simulink model "gm_sampleModel1552_5_sub"  (R2023a)
settings: Solver=VariableStepAuto  StartTime=0.0  StopTime=10.0  RelTol=1e-3
libraries: simulink x2
settings Model: Creator=user1  LastModifiedBy=user1
settings OptimizationCC: BlockReduction=off  ConditionallyExecuteInputs=off
settings DebuggingCC: InheritedTsInSrcMsg=none

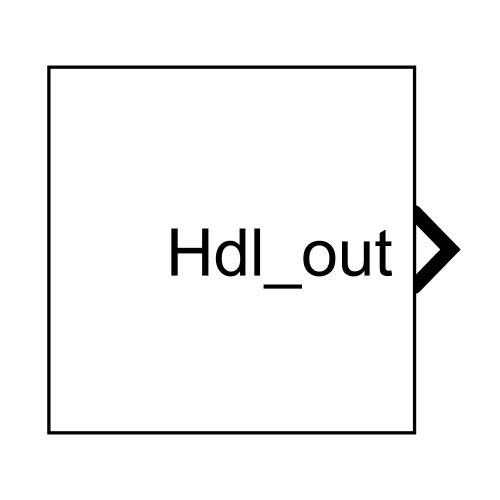
[thumbnail: Simulink's stored preview of the top-level diagram]
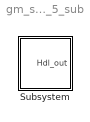
== system gm_sampleModel1552_5_sub ==
  Subsystem : Subsystem

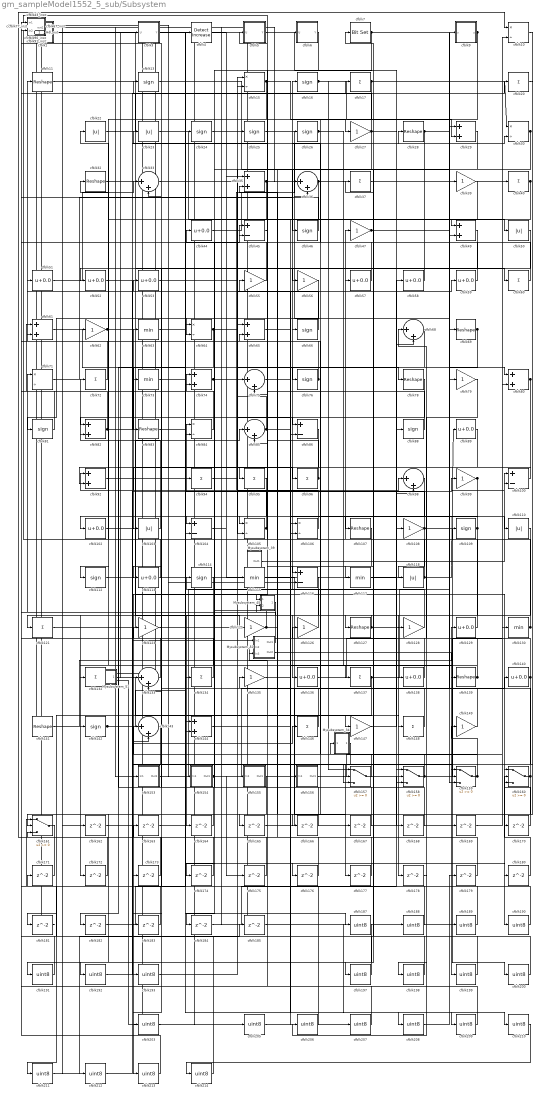
== system gm_sampleModel1552_5_sub/Subsystem ==
  Mysubsystem_34 : Subsystem
  Mysubsystem_39 : Subsystem
  Mysubsystem_45 : Subsystem
  Mysubsystem_50 : Subsystem
  Mysubsystem_51 : Subsystem
  cfblk1 : Subsystem  mask(Detect Fall Negative){vinit=double(0), InputProcessing=Elements as channels (sample based), OutDataTypeStr=uint8}
      mask prompts: vinit "Simulink:masks:InitialCondition_MP"; InputProcessing "Simulink:masks:InputProcessing_MP"; OutDataTypeStr "Simulink:masks:OutputDataType_MP"
      mask help: Simulink:masks:DetectFallNegative_MD
      mask init:
      | InputProcessing = 'Elements as channels (sample based)';
      | OutDataTypeStr = 'uint8';
      | vinit = double(0);
      mask TypeOptions InputProcessing: Simulink:masks:ColumnsAsChannelsFrameBased | Simulink:masks:ElementsAsChannelsSampleBased
      mask TypeOptions OutDataTypeStr: Simulink:masks:uint8 | Simulink:masks:boolean
      mask Display: fprintf('U < 0\n&  NOT\nU/z < 0')
  cfblk{10,15,30,64,71,84,105..106} (8 alike) : Product  Inputs=*/  OutDataTypeStr=uint8  RndMeth=Zero  SaturateOnIntegerOverflow=on
  cfblk{45,86,100,104,116} (5 alike) : Sum  Inputs=+-  OutDataTypeStr=uint8
  cfblk{44,51..53,57..59,89,102,113,129,136,138,140} (14 alike) : Bias  Bias=0.0  SaturateOnIntegerOverflow=off
  cfblk{22..23,50,103,110,118} (6 alike) : Abs  OutDataTypeStr=uint8  SaturateOnIntegerOverflow=off
  cfblk{11,28,32,69,78,83,107,127,139,141} (10 alike) : Reshape
  cfblk{27,39,47,55..56,62,79,99,108,123,125..126,128,135,147,149} (16 alike) : Gain  OutDataTypeStr=uint8
  cfblk{13,16,24..26,46,66,76,81,88,109,112,114,142} (14 alike) : Signum
  cfblk{63,73,115,117,130} (5 alike) : MinMax  OutDataTypeStr=uint8
  cfblk120_inst : Subsystem
  cfblk{17,20,37,40,60,72,94..96,121,132,134,137,146,148} (15 alike) : Sum  Inputs=+  OutDataTypeStr=uint8
  cfblk122_inst : Subsystem
  cfblk124_inst : Subsystem
  cfblk131_inst : Subsystem
  cfblk{33,36,68,75,85,98,133,143} (8 alike) : Sum  Inputs=|++  OutDataTypeStr=uint8
  cfblk{29,35,49,61,65,74,80,82,92,144} (10 alike) : Sum  OutDataTypeStr=uint8
  cfblk153 : Subsystem
  cfblk154 : Subsystem
  cfblk155 : Subsystem
  cfblk156 : Subsystem
  cfblk{157..161} (5 alike) : Switch  OutDataTypeStr=uint8  SaturateOnIntegerOverflow=off  InputSameDT=off
  cfblk{162..185} (24 alike) : Delay  SampleTime=1
  cfblk{187..193,197..200,203,205..214} (22 alike) : DataTypeConversion  OutDataTypeStr=uint8  SaturateOnIntegerOverflow=off  RndMeth=Floor
  cfblk18_inst : Subsystem
  cfblk21_inst : Subsystem
  cfblk3 : Subsystem  mask(Detect Rise Positive){vinit=double(0), InputProcessing=Elements as channels (sample based), OutDataTypeStr=uint8}
      mask prompts: vinit "Simulink:masks:InitialCondition_MP"; InputProcessing "Simulink:masks:InputProcessing_MP"; OutDataTypeStr "Simulink:masks:OutputDataType_MP"
      mask help: Simulink:masks:DetectRisePositive_MD
      mask init:
      | InputProcessing = 'Elements as channels (sample based)';
      | OutDataTypeStr = 'uint8';
      | vinit = double(0);
      mask TypeOptions InputProcessing: Simulink:masks:ColumnsAsChannelsFrameBased | Simulink:masks:ElementsAsChannelsSampleBased
      mask TypeOptions OutDataTypeStr: Simulink:masks:uint8 | Simulink:masks:boolean
      mask Display: fprintf('U > 0\n&  NOT\nU/z > 0')
  cfblk31_inst : Subsystem
  cfblk4 : simulink/Logic and Bit Operations/Detect Increase  vinit=0.0  OutDataTypeStr=uint8
      settings: LibrarySourceBlock=|
      | hdlsllib/Logic and Bit
      | Operations/Detect
      | Increase
  cfblk41_inst : Subsystem
  cfblk43_inst : Subsystem
  cfblk5 : Subsystem  mask(Detect Rise Nonnegative){vinit=double(0), InputProcessing=Elements as channels (sample based), OutDataTypeStr=uint8}
      mask prompts: vinit "Simulink:masks:InitialCondition_MP"; InputProcessing "Simulink:masks:InputProcessing_MP"; OutDataTypeStr "Simulink:masks:OutputDataType_MP"
      mask help: Simulink:masks:DetectRiseNonnegative_MD
      mask init:
      | InputProcessing = 'Elements as channels (sample based)';
      | OutDataTypeStr = 'uint8';
      | vinit = double(0);
      mask TypeOptions InputProcessing: Simulink:masks:ColumnsAsChannelsFrameBased | Simulink:masks:ElementsAsChannelsSampleBased
      mask TypeOptions OutDataTypeStr: Simulink:masks:uint8 | Simulink:masks:boolean
      mask Display: fprintf('U >= 0\n&  NOT\nU/z >= 0')
  cfblk6 : Subsystem  mask(Detect Rise Positive){vinit=double(0), InputProcessing=Elements as channels (sample based), OutDataTypeStr=uint8}
      mask prompts: vinit "Simulink:masks:InitialCondition_MP"; InputProcessing "Simulink:masks:InputProcessing_MP"; OutDataTypeStr "Simulink:masks:OutputDataType_MP"
      mask help: Simulink:masks:DetectRisePositive_MD
      mask init:
      | InputProcessing = 'Elements as channels (sample based)';
      | OutDataTypeStr = 'uint8';
      | vinit = double(0);
      mask TypeOptions InputProcessing: Simulink:masks:ColumnsAsChannelsFrameBased | Simulink:masks:ElementsAsChannelsSampleBased
      mask TypeOptions OutDataTypeStr: Simulink:masks:uint8 | Simulink:masks:boolean
      mask Display: fprintf('U > 0\n&  NOT\nU/z > 0')
  cfblk67_inst : Subsystem
  cfblk7 : simulink/Logic and Bit Operations/Bit Set  iBit=0
      settings: LibrarySourceBlock=|
      | hdlsllib/Logic and Bit
      | Operations/Bit Set
  cfblk77_inst : Subsystem
  cfblk8 : Constant  Value=0  OutDataTypeStr=uint8  SampleTime=1
  cfblk9 : Subsystem  mask(Compare To Zero){relop=<=, OutDataTypeStr=uint8, ZeroCross=on}
      mask prompts: relop "Simulink:masks:Operator_MP"; OutDataTypeStr "Simulink:masks:OutputDataType_MP"; ZeroCross "Simulink:masks:EnableZerocrossingDetection_MP"
      mask help: Simulink:masks:CompareToZero_MD
      mask init:
      | OutDataTypeStr = 'uint8';
      | ZeroCross = 'on';
      | blkName = 'sampleModel1552_5_sub/Subsystem/cfblk9';
      | relop = '<=';
      | setValue = 'fixdt(0, 8)';
      mask TypeOptions relop: == | ~= | < | <= | >= | >
      mask TypeOptions OutDataTypeStr: Simulink:masks:uint8 | Simulink:masks:boolean
      mask Callback ZeroCross: sl('zeroCrossEnable', gcbh);
      mask Display: disp([relop,' 0'])
  cfblk90_inst : Subsystem
  cfblk91_inst : Subsystem
  Hdl_out : Outport  OutDataTypeStr=uint8  SampleTime=1
  wires:
  Mysubsystem_34/1(Out1) -> cfblk177/1
  Mysubsystem_39/1(Out1) -> cfblk100/1
  Mysubsystem_45/1(Out1) -> cfblk172/1
  Mysubsystem_50/1(Out1) -> Mysubsystem_45/2(In2)
  Mysubsystem_50/2(Out2) -> cfblk199/1
  Mysubsystem_51/1(Out1) -> cfblk178/1
  cfblk1/1(Y) -> cfblk190/1
  cfblk10/1 -> cfblk160/1
  cfblk100/1 -> cfblk95/1
  cfblk102/1 -> cfblk84/1
  cfblk103/1 -> cfblk72/1
  cfblk104/1 -> cfblk35/1
  cfblk105/1 -> cfblk41_inst/1(in1), cfblk55/1, cfblk63/1
  cfblk106/1 -> cfblk53/1
  cfblk107/1 -> cfblk213/1
  cfblk108/1 -> cfblk200/1, cfblk118/1, cfblk100/2, cfblk84/2
  cfblk109/1 -> cfblk127/1, cfblk105/1, cfblk148/1
  cfblk11/1 -> cfblk168/1
  cfblk110/1 -> cfblk164/1
  cfblk112/1 -> cfblk125/1
  cfblk113/1 -> cfblk22/1
  cfblk114/1 -> cfblk142/1
  cfblk115/1 -> cfblk167/1
  cfblk116/1 -> cfblk136/1
  cfblk117/1 -> cfblk58/1
  cfblk118/1 -> cfblk89/1, cfblk47/1, Hdl_out/1
  cfblk120_inst/1(out1) -> cfblk188/1, cfblk162/1
  cfblk121/1 -> cfblk85/1
  cfblk122_inst/1(out1) -> cfblk141/1
  cfblk123/1 -> cfblk98/1
  cfblk124_inst/1(out1) -> cfblk205/1
  cfblk125/1 -> cfblk44/1, cfblk161/2
  cfblk126/1 -> cfblk16/1
  cfblk127/1 -> cfblk39/1, cfblk121/1
  cfblk128/1 -> cfblk114/1
  cfblk129/1 -> cfblk5/1(U)
  cfblk13/1 -> cfblk109/1
  cfblk130/1 -> cfblk91_inst/2(in2), cfblk74/1
  cfblk131_inst/1(out1) -> cfblk40/1
  cfblk132/1 -> cfblk3/1(U)
  cfblk133/1 -> cfblk120_inst/2(in2)
  cfblk134/1 -> cfblk123/1
  cfblk135/1 -> cfblk208/1
  cfblk136/1 -> cfblk68/2
  cfblk137/1 -> cfblk181/1, cfblk9/1(u)
  cfblk138/1 -> cfblk122_inst/2(in2)
  cfblk139/1 -> cfblk41_inst/2(in2), cfblk133/1, cfblk71/1
  cfblk140/1 -> cfblk68/1, cfblk173/1
  cfblk141/1 -> cfblk129/1
  cfblk142/1 -> cfblk193/1, cfblk4/1
  cfblk143/1 -> cfblk153/1(In1)
  cfblk144/1 -> cfblk106/1
  cfblk146/1 -> Mysubsystem_50/2(In2)
  cfblk147/1 -> cfblk108/1
  cfblk148/1 -> cfblk92/1
  cfblk149/1 -> cfblk126/1
  cfblk15/1 -> cfblk102/1, cfblk27/1
  cfblk153/1(Out1) -> cfblk88/1
  cfblk154/1(Out1) -> cfblk140/1, cfblk175/1, cfblk174/1
  cfblk155/1(Out1) -> cfblk192/1
  cfblk156/1(Out1) -> cfblk130/1
  cfblk157/1 -> cfblk66/1
  cfblk158/1 -> cfblk80/2, cfblk143/1
  cfblk159/1 -> cfblk149/1, Mysubsystem_34/1(In1)
  cfblk16/1 -> cfblk29/2, cfblk157/1
  cfblk160/1 -> cfblk67_inst/2(in2), cfblk211/1
  cfblk161/1 -> cfblk10/1
  cfblk162/1 -> cfblk143/2
  cfblk163/1 -> cfblk187/1
  cfblk164/1 -> cfblk33/2
  cfblk165/1 -> cfblk49/2
  cfblk166/1 -> cfblk35/2
  cfblk167/1 -> cfblk74/2
  cfblk168/1 -> cfblk82/2
  cfblk169/1 -> cfblk10/2
  cfblk17/1 -> cfblk86/1, cfblk30/1
  cfblk170/1 -> cfblk160/2
  cfblk171/1 -> cfblk131_inst/2(in2)
  cfblk172/1 -> cfblk21_inst/1(in1)
  cfblk173/1 -> cfblk161/3
  cfblk174/1 -> cfblk77_inst/1(in1)
  cfblk175/1 -> cfblk15/2
  cfblk176/1 -> cfblk65/2
  cfblk177/1 -> cfblk122_inst/1(in1)
  cfblk178/1 -> cfblk206/1
  cfblk179/1 -> cfblk67_inst/1(in1)
  cfblk18_inst/1(out1) -> cfblk212/1
  cfblk180/1 -> cfblk160/3
  cfblk181/1 -> cfblk1/1(U)
  cfblk182/1 -> cfblk104/2
  cfblk183/1 -> cfblk161/1
  cfblk184/1 -> cfblk158/2
  cfblk185/1 -> cfblk210/1
  cfblk187/1 -> cfblk191/1
  cfblk188/1 -> cfblk163/1
  cfblk189/1 -> cfblk131_inst/1(in1)
  cfblk190/1 -> cfblk90_inst/1(in1)
  cfblk191/1 -> cfblk90_inst/2(in2)
  cfblk192/1 -> cfblk99/1
  cfblk193/1 -> cfblk155/1(In1)
  cfblk197/1 -> cfblk21_inst/2(in2)
  cfblk198/1 -> cfblk37/1
  cfblk199/1 -> cfblk171/1
  cfblk20/1 -> cfblk170/1
  cfblk200/1 -> Mysubsystem_50/3(In3)
  cfblk203/1 -> Mysubsystem_51/2(In2)
  cfblk205/1 -> cfblk57/1
  cfblk206/1 -> cfblk124_inst/1(in1)
  cfblk207/1 -> cfblk124_inst/2(in2)
  cfblk208/1 -> cfblk179/1
  cfblk209/1 -> cfblk135/1
  cfblk21_inst/1(out1) -> cfblk207/1
  cfblk210/1 -> cfblk214/1
  cfblk211/1 -> cfblk185/1
  cfblk212/1 -> cfblk146/1
  cfblk213/1 -> cfblk18_inst/1(in1)
  cfblk214/1 -> cfblk18_inst/2(in2)
  cfblk22/1 -> cfblk17/1
  cfblk23/1 -> cfblk69/1
  cfblk24/1 -> cfblk25/1
  cfblk25/1 -> cfblk79/1
  cfblk26/1 -> cfblk138/1, cfblk60/1
  cfblk27/1 -> cfblk98/2, cfblk77_inst/2(in2), cfblk165/1
  cfblk28/1 -> cfblk50/1, cfblk184/1
  cfblk29/1 -> cfblk144/2
  cfblk3/1(Y) -> cfblk176/1
  cfblk30/1 -> cfblk46/1, cfblk157/3, cfblk105/2
  cfblk31_inst/1(out1) -> cfblk159/2
  cfblk32/1 -> cfblk56/1
  cfblk33/1 -> cfblk78/1
  cfblk35/1 -> cfblk36/2, cfblk112/1
  cfblk36/1 -> cfblk49/1, cfblk64/2
  cfblk37/1 -> cfblk197/1
  cfblk39/1 -> cfblk106/2
  cfblk4/1 -> Mysubsystem_51/1(In1)
  cfblk40/1 -> cfblk158/3, cfblk107/1
  cfblk41_inst/1(out1) -> cfblk43_inst/1(in1)
  cfblk43_inst/1(out1) -> cfblk116/2, cfblk115/1
  cfblk44/1 -> cfblk29/1
  cfblk45/1 -> Mysubsystem_45/1(In1)
  cfblk46/1 -> cfblk31_inst/1(in1)
  cfblk47/1 -> cfblk80/1, cfblk117/1
  cfblk49/1 -> cfblk113/1
  cfblk5/1(Y) -> cfblk158/1
  cfblk50/1 -> cfblk183/1
  cfblk51/1 -> cfblk33/1
  cfblk52/1 -> cfblk159/1
  cfblk53/1 -> cfblk75/1
  cfblk55/1 -> cfblk31_inst/2(in2)
  cfblk56/1 -> cfblk81/1
  cfblk57/1 -> cfblk26/1
  cfblk58/1 -> cfblk52/1
  cfblk59/1 -> cfblk43_inst/2(in2)
  cfblk6/1(Y) -> cfblk104/1
  cfblk60/1 -> cfblk7/1
  cfblk61/1 -> cfblk94/1
  cfblk62/1 -> Mysubsystem_50/1(In1), cfblk20/1
  cfblk63/1 -> cfblk144/1
  cfblk64/1 -> cfblk76/1, cfblk203/1
  cfblk65/1 -> cfblk139/1
  cfblk66/1 -> cfblk15/1
  cfblk67_inst/1(out1) -> cfblk24/1
  cfblk68/1 -> cfblk166/1
  cfblk69/1 -> cfblk83/1, cfblk182/1
  cfblk7/1 -> cfblk75/2, cfblk159/3
  cfblk71/1 -> cfblk36/1
  cfblk72/1 -> cfblk11/1
  cfblk73/1 -> cfblk209/1
  cfblk74/1 -> cfblk86/2, cfblk59/1
  cfblk75/1 -> cfblk110/1
  cfblk76/1 -> cfblk91_inst/1(in1), cfblk61/2, cfblk73/1
  cfblk77_inst/1(out1) -> cfblk154/1(In1), cfblk156/1(In1)
  cfblk78/1 -> cfblk82/1
  cfblk79/1 -> cfblk128/1
  cfblk8/1 -> cfblk71/2, cfblk6/1(U)
  cfblk80/1 -> cfblk92/2, cfblk133/2
  cfblk81/1 -> cfblk120_inst/1(in1)
  cfblk82/1 -> cfblk61/1, cfblk28/1, cfblk96/1
  cfblk83/1 -> cfblk147/1
  cfblk84/1 -> cfblk32/1
  cfblk85/1 -> cfblk65/1, cfblk180/1
  cfblk86/1 -> cfblk103/1
  cfblk88/1 -> cfblk51/1
  cfblk89/1 -> cfblk137/1
  cfblk9/1(y) -> cfblk85/2, cfblk116/1, cfblk64/1
  cfblk90_inst/1(out1) -> cfblk189/1
  cfblk91_inst/1(out1) -> cfblk62/1, cfblk169/1
  cfblk92/1 -> cfblk45/1
  cfblk94/1 -> cfblk30/2
  cfblk95/1 -> cfblk134/1
  cfblk96/1 -> cfblk45/2, cfblk23/1, cfblk13/1
  cfblk98/1 -> cfblk132/1
  cfblk99/1 -> cfblk198/1, cfblk157/2

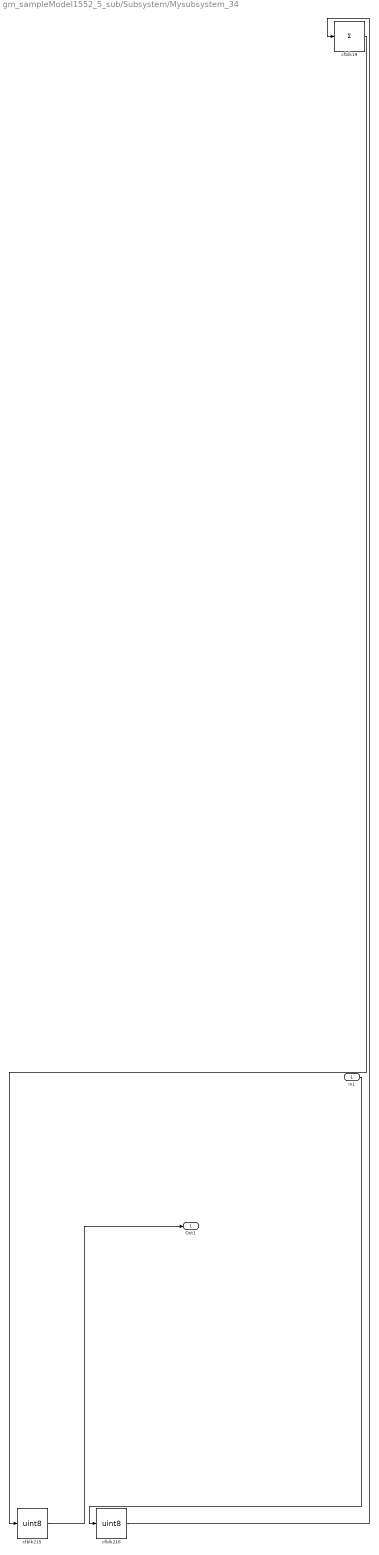
== system gm_sampleModel1552_5_sub/Subsystem/Mysubsystem_34 ==
  In1 : Inport  OutDataTypeStr=uint8  PortDimensions=1  SampleTime=1
  cfblk19 : Sum  Inputs=+
  cfblk215 : DataTypeConversion  OutDataTypeStr=uint8  SaturateOnIntegerOverflow=off  RndMeth=Floor
  cfblk216 : DataTypeConversion  OutDataTypeStr=uint8  SaturateOnIntegerOverflow=off  RndMeth=Floor
  Out1 : Outport  SampleTime=1
  wires:
  In1/1 -> cfblk216/1
  cfblk19/1 -> cfblk215/1
  cfblk215/1 -> Out1/1
  cfblk216/1 -> cfblk19/1

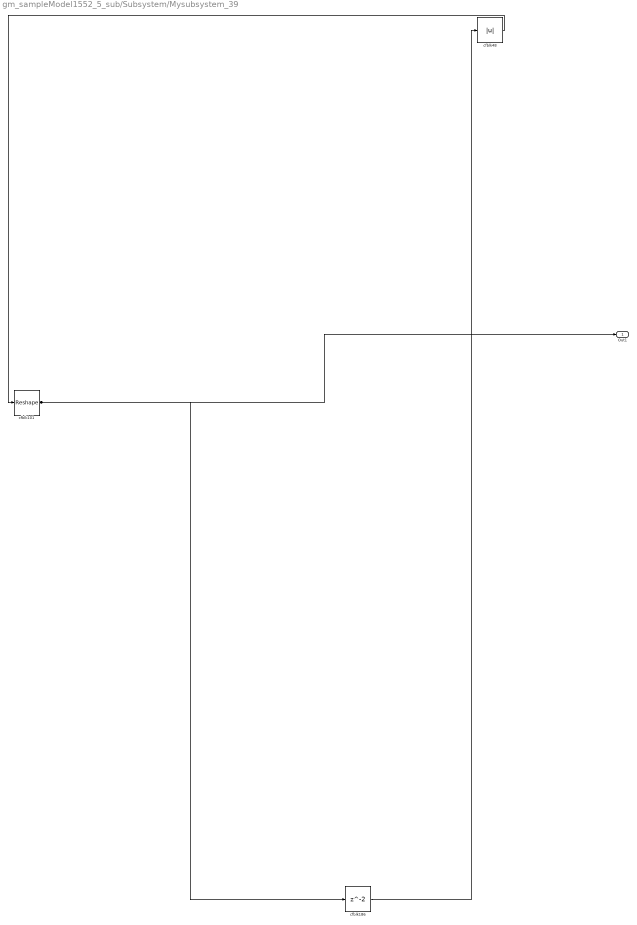
== system gm_sampleModel1552_5_sub/Subsystem/Mysubsystem_39 ==
  cfblk101 : Reshape
  cfblk186 : Delay  SampleTime=1
  cfblk48 : Abs  SaturateOnIntegerOverflow=off
  Out1 : Outport  SampleTime=1
  wires:
  cfblk101/1 -> cfblk186/1, Out1/1
  cfblk186/1 -> cfblk48/1
  cfblk48/1 -> cfblk101/1

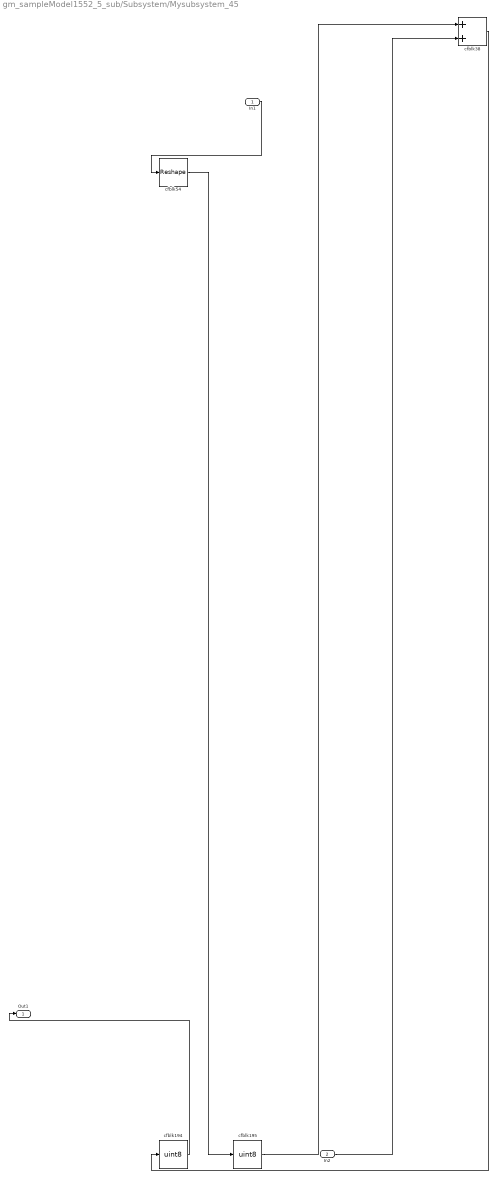
== system gm_sampleModel1552_5_sub/Subsystem/Mysubsystem_45 ==
  In1 : Inport  OutDataTypeStr=uint8  PortDimensions=1  SampleTime=1
  In2 : Inport  Port=2  OutDataTypeStr=uint8  PortDimensions=1  SampleTime=1
  cfblk194 : DataTypeConversion  OutDataTypeStr=uint8  SaturateOnIntegerOverflow=off  RndMeth=Floor
  cfblk195 : DataTypeConversion  OutDataTypeStr=uint8  SaturateOnIntegerOverflow=off  RndMeth=Floor
  cfblk38 : Sum
  cfblk54 : Reshape
  Out1 : Outport  SampleTime=1
  wires:
  In1/1 -> cfblk54/1
  In2/1 -> cfblk38/2
  cfblk194/1 -> Out1/1
  cfblk195/1 -> cfblk38/1
  cfblk38/1 -> cfblk194/1
  cfblk54/1 -> cfblk195/1

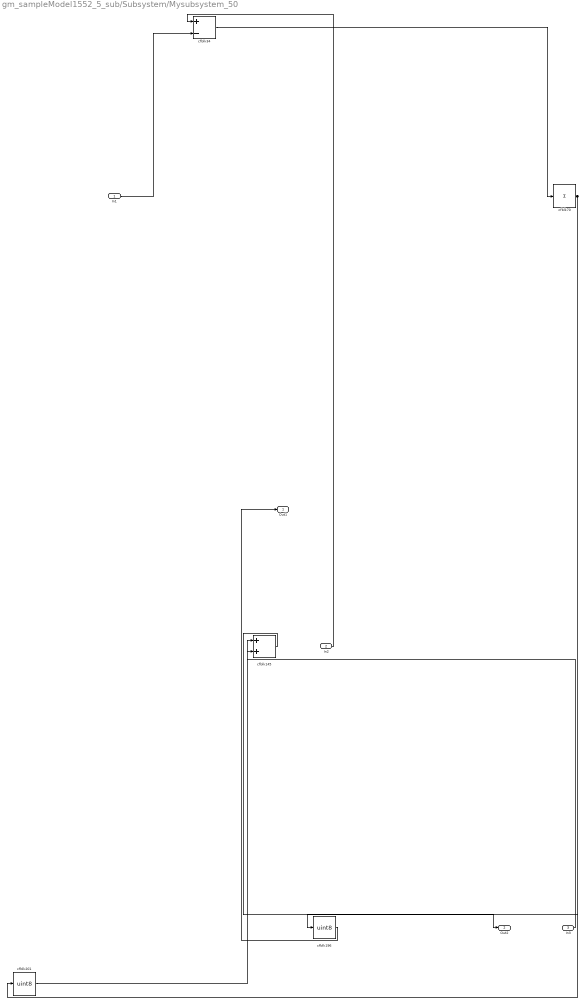
== system gm_sampleModel1552_5_sub/Subsystem/Mysubsystem_50 ==
  In1 : Inport  OutDataTypeStr=uint8  PortDimensions=1  SampleTime=1
  In2 : Inport  Port=2  OutDataTypeStr=uint8  PortDimensions=1  SampleTime=1
  In3 : Inport  Port=3  OutDataTypeStr=uint8  PortDimensions=1  SampleTime=1
  cfblk145 : Sum
  cfblk196 : DataTypeConversion  OutDataTypeStr=uint8  SaturateOnIntegerOverflow=off  RndMeth=Floor
  cfblk201 : DataTypeConversion  OutDataTypeStr=uint8  SaturateOnIntegerOverflow=off  RndMeth=Floor
  cfblk34 : Sum  Inputs=+-
  cfblk70 : Sum  Inputs=+
  Out1 : Outport  SampleTime=1
  Out2 : Outport  Port=2  SampleTime=1
  wires:
  In1/1 -> cfblk34/2
  In2/1 -> cfblk34/1
  In3/1 -> cfblk145/1
  cfblk145/1 -> Out2/1
  cfblk196/1 -> Out1/1
  cfblk201/1 -> cfblk145/2
  cfblk34/1 -> cfblk70/1
  cfblk70/1 -> cfblk201/1, cfblk196/1

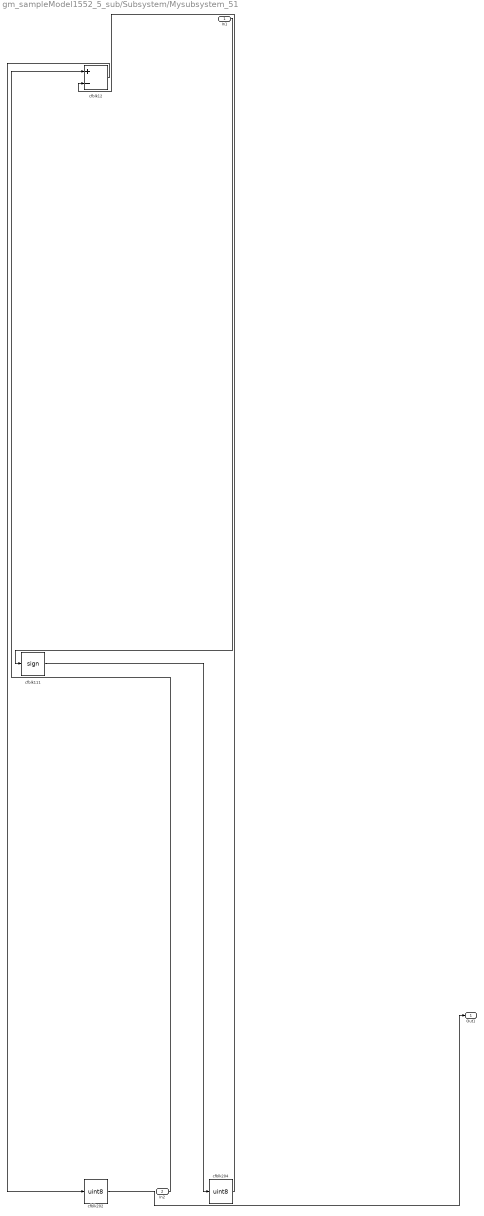
== system gm_sampleModel1552_5_sub/Subsystem/Mysubsystem_51 ==
  In1 : Inport  OutDataTypeStr=uint8  PortDimensions=1  SampleTime=1
  In2 : Inport  Port=2  OutDataTypeStr=uint8  PortDimensions=1  SampleTime=1
  cfblk111 : Signum
  cfblk12 : Sum  Inputs=+-
  cfblk202 : DataTypeConversion  OutDataTypeStr=uint8  SaturateOnIntegerOverflow=off  RndMeth=Floor
  cfblk204 : DataTypeConversion  OutDataTypeStr=uint8  SaturateOnIntegerOverflow=off  RndMeth=Floor
  Out1 : Outport  SampleTime=1
  wires:
  In1/1 -> cfblk111/1
  In2/1 -> cfblk12/1
  cfblk111/1 -> cfblk204/1
  cfblk12/1 -> cfblk202/1
  cfblk202/1 -> Out1/1
  cfblk204/1 -> cfblk12/2

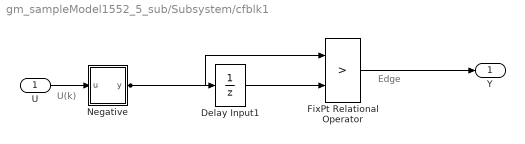
== system gm_sampleModel1552_5_sub/Subsystem/cfblk1 ==
  note: U(k)
  note: Edge
  U : Inport  OutDataTypeStr=uint8  SampleTime=1
  Delay Input1 : UnitDelay  Description=Store in Global RAM  DisableCoverage=on  InitialCondition=vinit  SampleTime=-1  HasFrameUpgradeWarning=on
  FixPt Relational Operator : RelationalOperator  Operator=>  OutDataTypeStr=fixdt(0, 8)  ZeroCross=off  InputSameDT=off
  Negative : Subsystem  mask(Compare To Zero){relop=<, OutDataTypeStr=boolean, ZeroCross=off}
      mask prompts: relop "Simulink:masks:Operator_MP"; OutDataTypeStr "Simulink:masks:OutputDataType_MP"; ZeroCross "Simulink:masks:EnableZerocrossingDetection_MP"
      mask help: Simulink:masks:CompareToZero_MD
      mask init:
      | OutDataTypeStr = 'boolean';
      | ZeroCross = 'off';
      | blkName = 'sampleModel1552_5_sub/Subsystem/cfblk1/Negative';
      | relop = '<';
      | setValue = 'boolean';
      mask TypeOptions relop: == | ~= | < | <= | >= | >
      mask TypeOptions OutDataTypeStr: Simulink:masks:uint8 | Simulink:masks:boolean
      mask Callback ZeroCross: sl('zeroCrossEnable', gcbh);
      mask Display: disp([relop,' 0'])
  Y : Outport  SampleTime=1
  wires:
  U/1 -> Negative/1(u)
  Delay Input1/1 -> FixPt Relational Operator/2
  FixPt Relational Operator/1 -> Y/1
  Negative/1(y) -> FixPt Relational Operator/1, Delay Input1/1

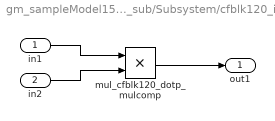
== system gm_sampleModel1552_5_sub/Subsystem/cfblk120_inst ==
  in1 : Inport  OutDataTypeStr=uint8  SampleTime=1
  in2 : Inport  Port=2  OutDataTypeStr=uint8  SampleTime=1
  mul_cfblk120_dotp_mulcomp : Product  Inputs=**  OutDataTypeStr=uint8  SampleTime=1
  out1 : Outport  OutDataTypeStr=uint8  SampleTime=1
  wires:
  in1/1 -> mul_cfblk120_dotp_mulcomp/1
  in2/1 -> mul_cfblk120_dotp_mulcomp/2
  mul_cfblk120_dotp_mulcomp/1 -> out1/1

== system gm_sampleModel1552_5_sub/Subsystem/cfblk122_inst ==
  in1 : Inport  OutDataTypeStr=uint8  SampleTime=1
  in2 : Inport  Port=2  OutDataTypeStr=uint8  SampleTime=1
  mul_cfblk122_dotp_mulcomp : Product  Inputs=**  OutDataTypeStr=uint8  SampleTime=1
  out1 : Outport  OutDataTypeStr=uint8  SampleTime=1
  wires:
  in1/1 -> mul_cfblk122_dotp_mulcomp/1
  in2/1 -> mul_cfblk122_dotp_mulcomp/2
  mul_cfblk122_dotp_mulcomp/1 -> out1/1

== system gm_sampleModel1552_5_sub/Subsystem/cfblk124_inst ==
  in1 : Inport  OutDataTypeStr=uint8  SampleTime=1
  in2 : Inport  Port=2  OutDataTypeStr=uint8  SampleTime=1
  mul_cfblk124_dotp_mulcomp : Product  Inputs=**  OutDataTypeStr=uint8  SampleTime=1
  out1 : Outport  OutDataTypeStr=uint8  SampleTime=1
  wires:
  in1/1 -> mul_cfblk124_dotp_mulcomp/1
  in2/1 -> mul_cfblk124_dotp_mulcomp/2
  mul_cfblk124_dotp_mulcomp/1 -> out1/1

== system gm_sampleModel1552_5_sub/Subsystem/cfblk131_inst ==
  in1 : Inport  OutDataTypeStr=uint8  SampleTime=1
  in2 : Inport  Port=2  OutDataTypeStr=uint8  SampleTime=1
  mul_cfblk131_dotp_mulcomp : Product  Inputs=**  OutDataTypeStr=uint8  SampleTime=1
  out1 : Outport  OutDataTypeStr=uint8  SampleTime=1
  wires:
  in1/1 -> mul_cfblk131_dotp_mulcomp/1
  in2/1 -> mul_cfblk131_dotp_mulcomp/2
  mul_cfblk131_dotp_mulcomp/1 -> out1/1

== system gm_sampleModel1552_5_sub/Subsystem/cfblk153 ==
  In1 : Inport  OutDataTypeStr=uint8  PortDimensions=1  SampleTime=1
  Out1 : Outport  SampleTime=1
  wires:
  In1/1 -> Out1/1

== system gm_sampleModel1552_5_sub/Subsystem/cfblk154 ==
  In1 : Inport  OutDataTypeStr=uint8  PortDimensions=1  SampleTime=1
  Out1 : Outport  SampleTime=1
  wires:
  In1/1 -> Out1/1

== system gm_sampleModel1552_5_sub/Subsystem/cfblk155 ==
  In1 : Inport  OutDataTypeStr=uint8  PortDimensions=1  SampleTime=1
  Out1 : Outport  SampleTime=1
  wires:
  In1/1 -> Out1/1

== system gm_sampleModel1552_5_sub/Subsystem/cfblk156 ==
  In1 : Inport  OutDataTypeStr=uint8  PortDimensions=1  SampleTime=1
  Out1 : Outport  SampleTime=1
  wires:
  In1/1 -> Out1/1

== system gm_sampleModel1552_5_sub/Subsystem/cfblk18_inst ==
  in1 : Inport  OutDataTypeStr=uint8  SampleTime=1
  in2 : Inport  Port=2  OutDataTypeStr=uint8  SampleTime=1
  mul_cfblk18_dotp_mulcomp : Product  Inputs=**  OutDataTypeStr=uint8  SampleTime=1
  out1 : Outport  OutDataTypeStr=uint8  SampleTime=1
  wires:
  in1/1 -> mul_cfblk18_dotp_mulcomp/1
  in2/1 -> mul_cfblk18_dotp_mulcomp/2
  mul_cfblk18_dotp_mulcomp/1 -> out1/1

== system gm_sampleModel1552_5_sub/Subsystem/cfblk21_inst ==
  in1 : Inport  OutDataTypeStr=uint8  SampleTime=1
  in2 : Inport  Port=2  OutDataTypeStr=uint8  SampleTime=1
  mul_cfblk21_dotp_mulcomp : Product  Inputs=**  OutDataTypeStr=uint8  SampleTime=1
  out1 : Outport  OutDataTypeStr=uint8  SampleTime=1
  wires:
  in1/1 -> mul_cfblk21_dotp_mulcomp/1
  in2/1 -> mul_cfblk21_dotp_mulcomp/2
  mul_cfblk21_dotp_mulcomp/1 -> out1/1

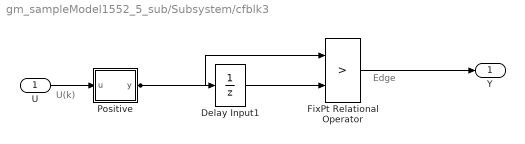
== system gm_sampleModel1552_5_sub/Subsystem/cfblk3 ==
  note: U(k)
  note: Edge
  U : Inport  OutDataTypeStr=uint8  SampleTime=1
  Delay Input1 : UnitDelay  Description=Store in Global RAM  DisableCoverage=on  InitialCondition=vinit  SampleTime=-1  HasFrameUpgradeWarning=on
  FixPt Relational Operator : RelationalOperator  Operator=>  OutDataTypeStr=fixdt(0, 8)  ZeroCross=off  InputSameDT=off
  Positive : Subsystem  mask(Compare To Zero){relop=>, OutDataTypeStr=boolean, ZeroCross=off}
      mask prompts: relop "Simulink:masks:Operator_MP"; OutDataTypeStr "Simulink:masks:OutputDataType_MP"; ZeroCross "Simulink:masks:EnableZerocrossingDetection_MP"
      mask help: Simulink:masks:CompareToZero_MD
      mask init:
      | OutDataTypeStr = 'boolean';
      | ZeroCross = 'off';
      | blkName = 'sampleModel1552_5_sub/Subsystem/cfblk3/Positive';
      | relop = '>';
      | setValue = 'boolean';
      mask TypeOptions relop: == | ~= | < | <= | >= | >
      mask TypeOptions OutDataTypeStr: Simulink:masks:uint8 | Simulink:masks:boolean
      mask Callback ZeroCross: sl('zeroCrossEnable', gcbh);
      mask Display: disp([relop,' 0'])
  Y : Outport  SampleTime=1
  wires:
  U/1 -> Positive/1(u)
  Delay Input1/1 -> FixPt Relational Operator/2
  FixPt Relational Operator/1 -> Y/1
  Positive/1(y) -> FixPt Relational Operator/1, Delay Input1/1

== system gm_sampleModel1552_5_sub/Subsystem/cfblk31_inst ==
  in1 : Inport  OutDataTypeStr=uint8  SampleTime=1
  in2 : Inport  Port=2  OutDataTypeStr=uint8  SampleTime=1
  mul_cfblk31_dotp_mulcomp : Product  Inputs=**  OutDataTypeStr=uint8  SampleTime=1
  out1 : Outport  OutDataTypeStr=uint8  SampleTime=1
  wires:
  in1/1 -> mul_cfblk31_dotp_mulcomp/1
  in2/1 -> mul_cfblk31_dotp_mulcomp/2
  mul_cfblk31_dotp_mulcomp/1 -> out1/1

== system gm_sampleModel1552_5_sub/Subsystem/cfblk41_inst ==
  in1 : Inport  OutDataTypeStr=uint8  SampleTime=1
  in2 : Inport  Port=2  OutDataTypeStr=uint8  SampleTime=1
  mul_cfblk41_dotp_mulcomp : Product  Inputs=**  OutDataTypeStr=uint8  SampleTime=1
  out1 : Outport  OutDataTypeStr=uint8  SampleTime=1
  wires:
  in1/1 -> mul_cfblk41_dotp_mulcomp/1
  in2/1 -> mul_cfblk41_dotp_mulcomp/2
  mul_cfblk41_dotp_mulcomp/1 -> out1/1

== system gm_sampleModel1552_5_sub/Subsystem/cfblk43_inst ==
  in1 : Inport  OutDataTypeStr=uint8  SampleTime=1
  in2 : Inport  Port=2  OutDataTypeStr=uint8  SampleTime=1
  mul_cfblk43_dotp_mulcomp : Product  Inputs=**  OutDataTypeStr=uint8  SampleTime=1
  out1 : Outport  OutDataTypeStr=uint8  SampleTime=1
  wires:
  in1/1 -> mul_cfblk43_dotp_mulcomp/1
  in2/1 -> mul_cfblk43_dotp_mulcomp/2
  mul_cfblk43_dotp_mulcomp/1 -> out1/1

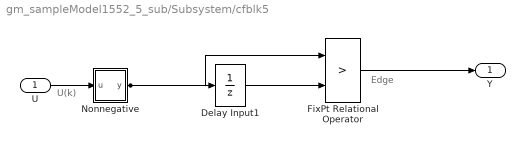
== system gm_sampleModel1552_5_sub/Subsystem/cfblk5 ==
  note: U(k)
  note: Edge
  U : Inport  OutDataTypeStr=uint8  SampleTime=1
  Delay Input1 : UnitDelay  Description=Store in Global RAM  DisableCoverage=on  InitialCondition=vinit  SampleTime=-1  HasFrameUpgradeWarning=on
  FixPt Relational Operator : RelationalOperator  Operator=>  OutDataTypeStr=fixdt(0, 8)  ZeroCross=off  InputSameDT=off
  Nonnegative : Subsystem  mask(Compare To Zero){relop=>=, OutDataTypeStr=boolean, ZeroCross=off}
      mask prompts: relop "Simulink:masks:Operator_MP"; OutDataTypeStr "Simulink:masks:OutputDataType_MP"; ZeroCross "Simulink:masks:EnableZerocrossingDetection_MP"
      mask help: Simulink:masks:CompareToZero_MD
      mask init:
      | OutDataTypeStr = 'boolean';
      | ZeroCross = 'off';
      | blkName = 'sampleModel1552_5_sub/Subsystem/cfblk5/Nonnegative';
      | relop = '>=';
      | setValue = 'boolean';
      mask TypeOptions relop: == | ~= | < | <= | >= | >
      mask TypeOptions OutDataTypeStr: Simulink:masks:uint8 | Simulink:masks:boolean
      mask Callback ZeroCross: sl('zeroCrossEnable', gcbh);
      mask Display: disp([relop,' 0'])
  Y : Outport  SampleTime=1
  wires:
  U/1 -> Nonnegative/1(u)
  Delay Input1/1 -> FixPt Relational Operator/2
  FixPt Relational Operator/1 -> Y/1
  Nonnegative/1(y) -> FixPt Relational Operator/1, Delay Input1/1

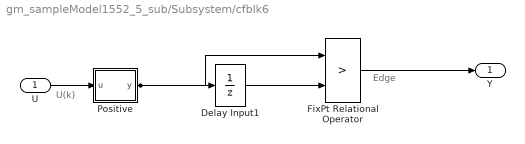
== system gm_sampleModel1552_5_sub/Subsystem/cfblk6 ==
  note: U(k)
  note: Edge
  U : Inport  OutDataTypeStr=uint8  SampleTime=1
  Delay Input1 : UnitDelay  Description=Store in Global RAM  DisableCoverage=on  InitialCondition=vinit  SampleTime=-1  HasFrameUpgradeWarning=on
  FixPt Relational Operator : RelationalOperator  Operator=>  OutDataTypeStr=fixdt(0, 8)  ZeroCross=off  InputSameDT=off
  Positive : Subsystem  mask(Compare To Zero){relop=>, OutDataTypeStr=boolean, ZeroCross=off}
      mask prompts: relop "Simulink:masks:Operator_MP"; OutDataTypeStr "Simulink:masks:OutputDataType_MP"; ZeroCross "Simulink:masks:EnableZerocrossingDetection_MP"
      mask help: Simulink:masks:CompareToZero_MD
      mask init:
      | OutDataTypeStr = 'boolean';
      | ZeroCross = 'off';
      | blkName = 'sampleModel1552_5_sub/Subsystem/cfblk6/Positive';
      | relop = '>';
      | setValue = 'boolean';
      mask TypeOptions relop: == | ~= | < | <= | >= | >
      mask TypeOptions OutDataTypeStr: Simulink:masks:uint8 | Simulink:masks:boolean
      mask Callback ZeroCross: sl('zeroCrossEnable', gcbh);
      mask Display: disp([relop,' 0'])
  Y : Outport  SampleTime=1
  wires:
  U/1 -> Positive/1(u)
  Delay Input1/1 -> FixPt Relational Operator/2
  FixPt Relational Operator/1 -> Y/1
  Positive/1(y) -> FixPt Relational Operator/1, Delay Input1/1

== system gm_sampleModel1552_5_sub/Subsystem/cfblk67_inst ==
  in1 : Inport  OutDataTypeStr=uint8  SampleTime=1
  in2 : Inport  Port=2  OutDataTypeStr=uint8  SampleTime=1
  mul_cfblk67_dotp_mulcomp : Product  Inputs=**  OutDataTypeStr=uint8  SampleTime=1
  out1 : Outport  OutDataTypeStr=uint8  SampleTime=1
  wires:
  in1/1 -> mul_cfblk67_dotp_mulcomp/1
  in2/1 -> mul_cfblk67_dotp_mulcomp/2
  mul_cfblk67_dotp_mulcomp/1 -> out1/1

== system gm_sampleModel1552_5_sub/Subsystem/cfblk77_inst ==
  in1 : Inport  OutDataTypeStr=uint8  SampleTime=1
  in2 : Inport  Port=2  OutDataTypeStr=uint8  SampleTime=1
  mul_cfblk77_dotp_mulcomp : Product  Inputs=**  OutDataTypeStr=uint8  SampleTime=1
  out1 : Outport  OutDataTypeStr=uint8  SampleTime=1
  wires:
  in1/1 -> mul_cfblk77_dotp_mulcomp/1
  in2/1 -> mul_cfblk77_dotp_mulcomp/2
  mul_cfblk77_dotp_mulcomp/1 -> out1/1

== system gm_sampleModel1552_5_sub/Subsystem/cfblk9 ==
  u : Inport  OutDataTypeStr=uint8  SampleTime=1
  Compare : RelationalOperator  Operator=<=  OutDataTypeStr=fixdt(0, 8)
  Constant : Constant  DisableCoverage=on  Value=0  OutDataTypeStr=Inherit: Inherit via back propagation  SampleTime=-1  PreserveConstantTs=on
  y : Outport  SampleTime=1
  wires:
  u/1 -> Compare/1
  Compare/1 -> y/1
  Constant/1 -> Compare/2

== system gm_sampleModel1552_5_sub/Subsystem/cfblk90_inst ==
  in1 : Inport  OutDataTypeStr=uint8  SampleTime=1
  in2 : Inport  Port=2  OutDataTypeStr=uint8  SampleTime=1
  mul_cfblk90_dotp_mulcomp : Product  Inputs=**  OutDataTypeStr=uint8  SampleTime=1
  out1 : Outport  OutDataTypeStr=uint8  SampleTime=1
  wires:
  in1/1 -> mul_cfblk90_dotp_mulcomp/1
  in2/1 -> mul_cfblk90_dotp_mulcomp/2
  mul_cfblk90_dotp_mulcomp/1 -> out1/1

== system gm_sampleModel1552_5_sub/Subsystem/cfblk91_inst ==
  in1 : Inport  OutDataTypeStr=uint8  SampleTime=1
  in2 : Inport  Port=2  OutDataTypeStr=uint8  SampleTime=1
  mul_cfblk91_dotp_mulcomp : Product  Inputs=**  OutDataTypeStr=uint8  SampleTime=1
  out1 : Outport  OutDataTypeStr=uint8  SampleTime=1
  wires:
  in1/1 -> mul_cfblk91_dotp_mulcomp/1
  in2/1 -> mul_cfblk91_dotp_mulcomp/2
  mul_cfblk91_dotp_mulcomp/1 -> out1/1

== system gm_sampleModel1552_5_sub/Subsystem/cfblk1/Negative ==
  u : Inport  OutDataTypeStr=uint8  SampleTime=1
  Compare : RelationalOperator  Operator=<  OutDataTypeStr=boolean  ZeroCross=off
  Constant : Constant  DisableCoverage=on  Value=0  OutDataTypeStr=Inherit: Inherit via back propagation  SampleTime=-1  PreserveConstantTs=on
  y : Outport  SampleTime=1
  wires:
  u/1 -> Compare/1
  Compare/1 -> y/1
  Constant/1 -> Compare/2

== system gm_sampleModel1552_5_sub/Subsystem/cfblk3/Positive ==
  u : Inport  OutDataTypeStr=uint8  SampleTime=1
  Compare : RelationalOperator  Operator=>  OutDataTypeStr=boolean  ZeroCross=off
  Constant : Constant  DisableCoverage=on  Value=0  OutDataTypeStr=Inherit: Inherit via back propagation  SampleTime=-1  PreserveConstantTs=on
  y : Outport  SampleTime=1
  wires:
  u/1 -> Compare/1
  Compare/1 -> y/1
  Constant/1 -> Compare/2

== system gm_sampleModel1552_5_sub/Subsystem/cfblk5/Nonnegative ==
  u : Inport  OutDataTypeStr=uint8  SampleTime=1
  Compare : RelationalOperator  OutDataTypeStr=boolean  ZeroCross=off
  Constant : Constant  DisableCoverage=on  Value=0  OutDataTypeStr=Inherit: Inherit via back propagation  SampleTime=-1  PreserveConstantTs=on
  y : Outport  SampleTime=1
  wires:
  u/1 -> Compare/1
  Compare/1 -> y/1
  Constant/1 -> Compare/2

== system gm_sampleModel1552_5_sub/Subsystem/cfblk6/Positive ==
  u : Inport  OutDataTypeStr=uint8  SampleTime=1
  Compare : RelationalOperator  Operator=>  OutDataTypeStr=boolean  ZeroCross=off
  Constant : Constant  DisableCoverage=on  Value=0  OutDataTypeStr=Inherit: Inherit via back propagation  SampleTime=-1  PreserveConstantTs=on
  y : Outport  SampleTime=1
  wires:
  u/1 -> Compare/1
  Compare/1 -> y/1
  Constant/1 -> Compare/2
